simulink model "slDxl_Ex"  (R2021a)
settings: Solver=VariableStepAuto  StartTime=0.0  StopTime=inf  RelTol=1e-3
libraries: slDxl_lib x10
settings Model: Creator=jeihunl  LastModifiedBy=johnc
settings SolverCC: AlgebraicLoopSolver=TrustRegion
settings DataIOCC: ReturnWorkspaceOutputs=off
settings DebuggingCC: SFMachineParentedDataDiag=warning  ArithmeticOperatorsInVariantConditions=warning
settings SFSimCC: SimCustomHeaderCode="#include \"dynamixel_sdk.h\""  SimUserLibraries=dxl_x64_c.lib  SimUseLocalCustomCode=off  SimParseCustomCode=off  CustomCodeUndefinedFunction=UseInterfaceOnly
settings SFSimCC: SimUserIncludeDirs=|
  | C:\Users\johnc\OneDrive\Documentos\DYNAMIXEL\DynamixelSDK-3.7.51\c\include\dynamixel_sdk\
  | C:\Users\johnc\OneDrive\Documentos\DYNAMIXEL\DynamixelSDK-3.7.51\c\build\win64\output\
  | C:\Users\johnc\OneDrive\Documentos\DYNAMIXEL\DynamixelSDK-3.7.51\c\src\dynamixel_sdk\
settings SFSimCC: SimUserDefines=|
  | _WIN32
  | _WIN64
  | _cplusplus
  | size_t=unsigned __int64
  | size_t=unsigned in
settings RTWCC: RTWUseLocalCustomCode=off
settings CodeAppCC: StateflowObjectComments=on

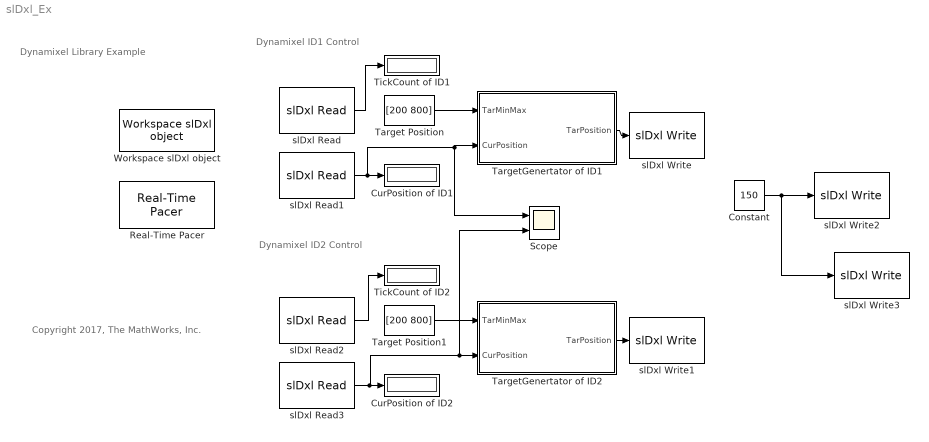
== system slDxl_Ex ==
  note: Dynamixel Library Example
  note: Copyright 2017, The MathWorks, Inc.
  note: Dynamixel ID2 Control
  note: Dynamixel ID1 Control
  Constant : Constant  Value=150
  CurPosition of ID1 : Display
  CurPosition of ID2 : Display
  Real-Time Pacer : slDxl_lib/Real-Time Pacer  simTimePerRealTime=1
  Scope : Scope  NumInputPorts=2
  Target Position : Constant  Value=[200 800]
  Target Position1 : Constant  Value=[200 800]
  TargetGenertator of ID1 : Stateflow chart  TreatAsAtomicUnit=on
  TargetGenertator of ID2 : Stateflow chart  TreatAsAtomicUnit=on
  TickCount of ID1 : Display
  TickCount of ID2 : Display
  Workspace slDxl object : slDxl_lib/Workspace slDxl object  slDxlVarName=Existing Object Handle #1  workspaceVarName=myDxl
  slDxl Read : slDxl_lib/slDxl Read  slDxlObject=Existing Object Handle #1  DXL_ID=1  DXL_ADDR=38  DXL_READ_SIZE=2  sampleT=Ts
  slDxl Read1 : slDxl_lib/slDxl Read  slDxlObject=Existing Object Handle #1  DXL_ID=1  DXL_ADDR=36  DXL_READ_SIZE=2  sampleT=Ts
  slDxl Read2 : slDxl_lib/slDxl Read  slDxlObject=Existing Object Handle #1  DXL_ID=2  DXL_ADDR=38  DXL_READ_SIZE=2  sampleT=Ts
  slDxl Read3 : slDxl_lib/slDxl Read  slDxlObject=Existing Object Handle #1  DXL_ID=2  DXL_ADDR=36  DXL_READ_SIZE=2  sampleT=Ts
  slDxl Write : slDxl_lib/slDxl Write  slDxlObject=Existing Object Handle #1  DXL_ID=1  DXL_ADDR=30  DXL_WRITE_SIZE=2  sampleT=Ts
  slDxl Write1 : slDxl_lib/slDxl Write  slDxlObject=Existing Object Handle #1  DXL_ID=2  DXL_ADDR=30  DXL_WRITE_SIZE=2  sampleT=Ts
  slDxl Write2 : slDxl_lib/slDxl Write  slDxlObject=Existing Object Handle #1  DXL_ID=1  DXL_ADDR=32  DXL_WRITE_SIZE=2  sampleT=Ts
  slDxl Write3 : slDxl_lib/slDxl Write  slDxlObject=Existing Object Handle #1  DXL_ID=2  DXL_ADDR=32  DXL_WRITE_SIZE=2  sampleT=Ts
  wires:
  slDxl Read/1 -> TickCount of ID1/1
  slDxl Read1/1 -> CurPosition of ID1/1, Scope/1, TargetGenertator of ID1/2(CurPosition)
  Target Position/1 -> TargetGenertator of ID1/1(TarMinMax)
  TargetGenertator of ID1/1(TarPosition) -> slDxl Write/1
  slDxl Read2/1 -> TickCount of ID2/1
  TargetGenertator of ID2/1(TarPosition) -> slDxl Write1/1
  Target Position1/1 -> TargetGenertator of ID2/1(TarMinMax)
  slDxl Read3/1 -> Scope/2, TargetGenertator of ID2/2(CurPosition), CurPosition of ID2/1
  Constant/1 -> slDxl Write3/1, slDxl Write2/1

== stateflow chart slDxl_Ex/TargetGenertator of ID2 ==
  state MinTarget
    en:
    TarPosition = TarMinMax(1);
  state CheckPosition
    en:
    Thres = 10;
  state MaxTarget
    en:
    TarPosition = TarMinMax(2);
  (default) -> CheckPosition
  (junction 19) -> MinTarget [order 1] : [CurPosition < 1024]
  MaxTarget -> MinTarget : [abs(TarMinMax(2)-CurPosition) < Thres]
  MinTarget -> MaxTarget : [abs(TarMinMax(1)-CurPosition) < Thres]
  CheckPosition -> (junction 19)
  (junction 19) -> MaxTarget [order 2]
  data: TarMinMax input; CurPosition input; TarPosition output; Thres local

== stateflow chart slDxl_Ex/TargetGenertator of ID1 ==
  state MinTarget
    en:
    TarPosition = TarMinMax(1);
  state CheckPosition
    en:
    Thres = 10;
  state MaxTarget
    en:
    TarPosition = TarMinMax(2);
  (default) -> CheckPosition
  (junction 19) -> MinTarget [order 1] : [CurPosition < TarMinMax(2)/2]
  MaxTarget -> MinTarget : [abs(TarMinMax(2)-CurPosition) < Thres]
  MinTarget -> MaxTarget : [abs(TarMinMax(1)-CurPosition) < Thres]
  CheckPosition -> (junction 19)
  (junction 19) -> MaxTarget [order 2]
  data: TarMinMax input; CurPosition input; TarPosition output; Thres local
